simulink model "siso_example_ublf_blf_bs"  (R2021a)
settings: Solver=ode4  StartTime=0.0  StopTime=1.5  FixedStep=0.001  RelTol=1e-3
model workspace (MAT data in the model file):
  scale_start = Simulink.Signal
  scale_start.DataType = 'double'
  scale_start.Dimensions = 1
  scale_start.DimensionsMode = 'auto'
  scale_start.Complexity = 'auto'
  scale_start.SampleTime = 0
  scale_start.SamplingMode = 'auto'
  scale_start.InitialValue = '1'
libraries: simulink x2
settings Model: OrderedModelArguments=off  Creator=14244039  LastModifiedBy=14244039

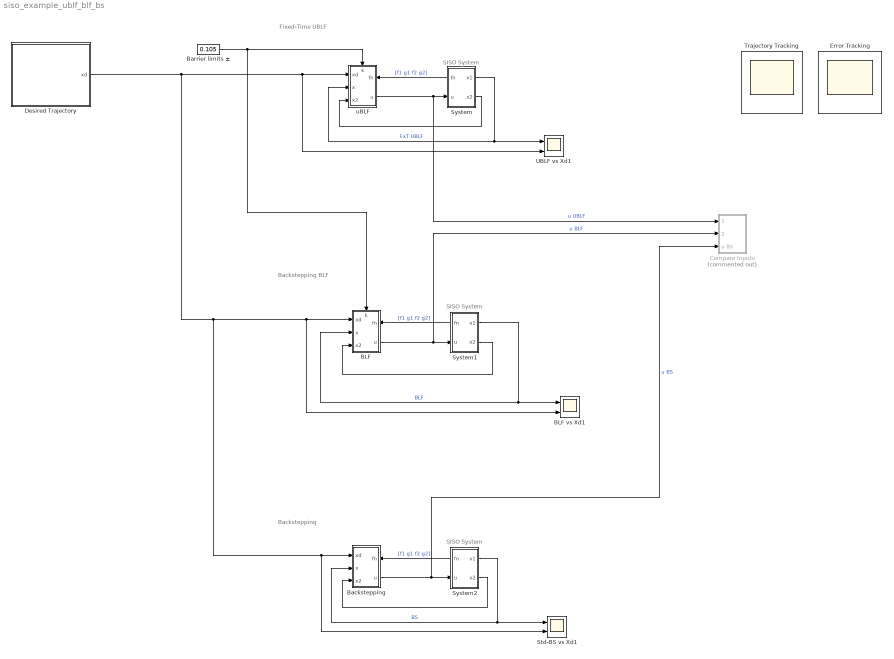
== system siso_example_ublf_blf_bs ==
  note: SISO System
  note: Backstepping
  note: Backstepping BLF
  note: Fixed-Time UBLF
  note: SISO System
  note: SISO System
  BLF : Subsystem
      settings: PortSchema="{\"entries\":[{\"content\":{\"sides\":[{\"content\":{\"connectorIds\":[\"In1\",\"In2\",\"In3\"]},\"type\":\"ConnectorPlacement.EquallySpacedRectSide\",\"uuid\":\"d2f7d382-6195-45e8-bd6d-6d057452a9ba\"},{\"content\":{\"connectorIds\":[\"In5\",\"Out1\"],\"side\":\"RIGHT\"},\"type\":\"ConnectorPlacement.EquallySpacedRectSide\",\"uuid\":\"a1535a06-1066-4f88-a239-6dd18a46e73c\"},{\"content\":{\"connectorIds\":[\"In4\"],\"side\":\"TOP\"},\"type\":\"ConnectorPlacement.EquallySpacedRectSide\",\"uuid\":\"b65ca63e-d25a-45d6-8018-31a25176dac1\"}]},\"type\":\"ConnectorPlacement.EquallySpacedConnector\",\"uuid\":\"280ac837-5d25-45ee-8f8e-187f8883864d\"}],\"packageUris\":[\"http://schema.mathworks.com/mf0/Connector/R2020b\"],\"version\":\"1.0\"}"
  BLF vs Xd1 : Scope  NumInputPorts=2
  Backstepping : Subsystem
      settings: PortSchema="{\"entries\":[{\"content\":{\"sides\":[{\"content\":{\"connectorIds\":[\"In1\",\"In2\",\"In3\"]},\"type\":\"ConnectorPlacement.EquallySpacedRectSide\",\"uuid\":\"d2f7d382-6195-45e8-bd6d-6d057452a9ba\"},{\"content\":{\"connectorIds\":[\"In4\",\"Out1\"],\"side\":\"RIGHT\"},\"type\":\"ConnectorPlacement.EquallySpacedRectSide\",\"uuid\":\"a1535a06-1066-4f88-a239-6dd18a46e73c\"},{\"content\":{\"connectorIds\":[],\"side\":\"TOP\"},\"type\":\"ConnectorPlacement.EquallySpacedRectSide\",\"uuid\":\"b65ca63e-d25a-45d6-8018-31a25176dac1\"}]},\"type\":\"ConnectorPlacement.EquallySpacedConnector\",\"uuid\":\"280ac837-5d25-45ee-8f8e-187f8883864d\"}],\"packageUris\":[\"http://schema.mathworks.com/mf0/Connector/R2020b\"],\"version\":\"1.0\"}"
  Barrier limits ± : Constant  Value=0.105
  Compare Inputs : Subsystem  Commented=on
  Desired Trajectory : Subsystem
  Error Tracking : Scope
      settings: Floating=on
  Std-BS vs Xd1 : Scope  NumInputPorts=2
  System : Subsystem
      settings: PortSchema="{\"entries\":[{\"content\":{\"sides\":[{\"content\":{\"connectorIds\":[\"Out3\",\"In1\"]},\"type\":\"ConnectorPlacement.EquallySpacedRectSide\",\"uuid\":\"44a46657-7d00-4f6d-80a4-fbe778e41b73\"},{\"content\":{\"connectorIds\":[\"Out1\",\"Out2\"],\"side\":\"RIGHT\"},\"type\":\"ConnectorPlacement.EquallySpacedRectSide\",\"uuid\":\"1134a23b-2977-450f-b075-fdef5e2c40fa\"},{\"content\":{\"connectorIds\":[],\"side\":\"TOP\"},\"type\":\"ConnectorPlacement.EquallySpacedRectSide\",\"uuid\":\"dbd99adc-543a-4e22-b7a4-6b9f86b8ed0c\"}]},\"type\":\"ConnectorPlacement.EquallySpacedConnector\",\"uuid\":\"979c4d4e-bab9-42b7-bb8f-441469f19c5c\"}],\"packageUris\":[\"http://schema.mathworks.com/mf0/Connector/R2020b\"],\"version\":\"1.0\"}"
  System1 : Subsystem
      settings: PortSchema="{\"entries\":[{\"content\":{\"sides\":[{\"content\":{\"connectorIds\":[\"Out3\",\"In1\"]},\"type\":\"ConnectorPlacement.EquallySpacedRectSide\",\"uuid\":\"44a46657-7d00-4f6d-80a4-fbe778e41b73\"},{\"content\":{\"connectorIds\":[\"Out1\",\"Out2\"],\"side\":\"RIGHT\"},\"type\":\"ConnectorPlacement.EquallySpacedRectSide\",\"uuid\":\"1134a23b-2977-450f-b075-fdef5e2c40fa\"},{\"content\":{\"connectorIds\":[],\"side\":\"TOP\"},\"type\":\"ConnectorPlacement.EquallySpacedRectSide\",\"uuid\":\"dbd99adc-543a-4e22-b7a4-6b9f86b8ed0c\"}]},\"type\":\"ConnectorPlacement.EquallySpacedConnector\",\"uuid\":\"979c4d4e-bab9-42b7-bb8f-441469f19c5c\"}],\"packageUris\":[\"http://schema.mathworks.com/mf0/Connector/R2020b\"],\"version\":\"1.0\"}"
  System2 : Subsystem
      settings: PortSchema="{\"entries\":[{\"content\":{\"sides\":[{\"content\":{\"connectorIds\":[\"Out3\",\"In1\"]},\"type\":\"ConnectorPlacement.EquallySpacedRectSide\",\"uuid\":\"44a46657-7d00-4f6d-80a4-fbe778e41b73\"},{\"content\":{\"connectorIds\":[\"Out1\",\"Out2\"],\"side\":\"RIGHT\"},\"type\":\"ConnectorPlacement.EquallySpacedRectSide\",\"uuid\":\"1134a23b-2977-450f-b075-fdef5e2c40fa\"},{\"content\":{\"connectorIds\":[],\"side\":\"TOP\"},\"type\":\"ConnectorPlacement.EquallySpacedRectSide\",\"uuid\":\"dbd99adc-543a-4e22-b7a4-6b9f86b8ed0c\"}]},\"type\":\"ConnectorPlacement.EquallySpacedConnector\",\"uuid\":\"979c4d4e-bab9-42b7-bb8f-441469f19c5c\"}],\"packageUris\":[\"http://schema.mathworks.com/mf0/Connector/R2020b\"],\"version\":\"1.0\"}"
  Trajectory Tracking : Scope
      settings: Floating=on
  UBLF vs Xd1 : Scope  NumInputPorts=2
  uBLF : Subsystem
      settings: PortSchema="{\"entries\":[{\"content\":{\"sides\":[{\"content\":{\"connectorIds\":[\"In1\",\"In2\",\"In3\"]},\"type\":\"ConnectorPlacement.EquallySpacedRectSide\",\"uuid\":\"d2f7d382-6195-45e8-bd6d-6d057452a9ba\"},{\"content\":{\"connectorIds\":[\"In5\",\"Out1\"],\"side\":\"RIGHT\"},\"type\":\"ConnectorPlacement.EquallySpacedRectSide\",\"uuid\":\"a1535a06-1066-4f88-a239-6dd18a46e73c\"},{\"content\":{\"connectorIds\":[\"In4\"],\"side\":\"TOP\"},\"type\":\"ConnectorPlacement.EquallySpacedRectSide\",\"uuid\":\"b65ca63e-d25a-45d6-8018-31a25176dac1\"}]},\"type\":\"ConnectorPlacement.EquallySpacedConnector\",\"uuid\":\"280ac837-5d25-45ee-8f8e-187f8883864d\"}],\"packageUris\":[\"http://schema.mathworks.com/mf0/Connector/R2020b\"],\"version\":\"1.0\"}"
  wires:
  System/1(x1) -> uBLF/2(x), UBLF vs Xd1/1  "FxT UBLF"
  System/2(x2) -> uBLF/3(x2)
  System/3(fn) -> uBLF/5(fn)  "[f1 g1 f2 g2]"
  uBLF/1(u) -> Compare Inputs/1(u UBLF), System/1(u)  "u UBLF"
  System1/3(fn) -> BLF/5(fn)  "[f1 g1 f2 g2]"
  BLF/1(u) -> Compare Inputs/2(u ABLF), System1/1(u)  "u BLF"
  System1/1(x1) -> BLF vs Xd1/1, BLF/2(x)  "BLF"
  System1/2(x2) -> BLF/3(x2)
  System2/1(x1) -> Backstepping/2(x), Std-BS vs Xd1/1  "BS"
  System2/2(x2) -> Backstepping/3(x2)
  Desired Trajectory/1(xd) -> uBLF/1(xd), UBLF vs Xd1/2, BLF/1(xd), BLF vs Xd1/2, Std-BS vs Xd1/2, Backstepping/1(xd)
  System2/3(fn) -> Backstepping/4(fn)  "[f1 g1 f2 g2]"
  Backstepping/1(u) -> Compare Inputs/3(u BS), System2/1(u)  "u BS"
  Barrier limits ±/1 -> BLF/4(k), uBLF/4(k)

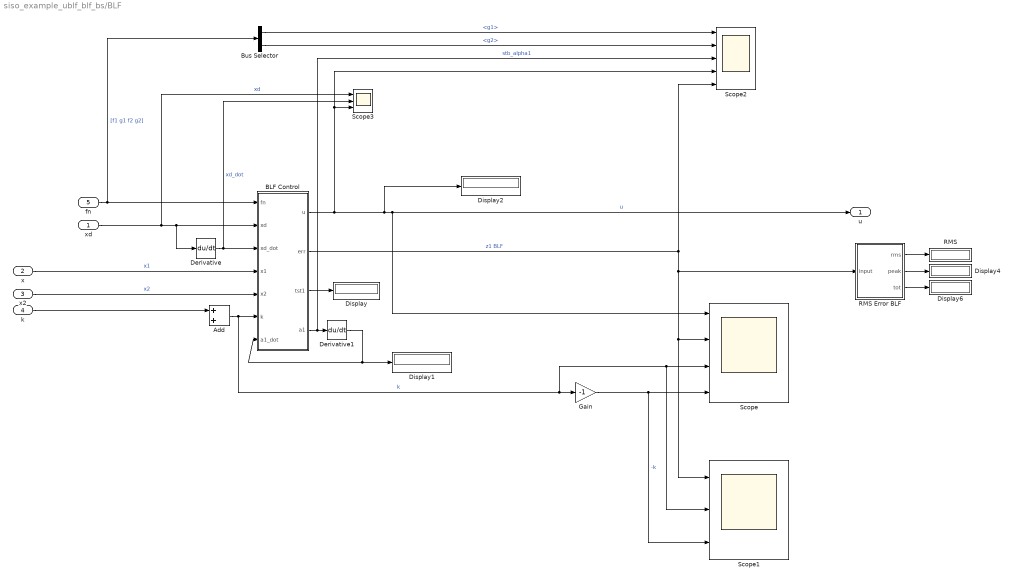
== system siso_example_ublf_blf_bs/BLF ==
  xd : Inport
  x : Inport  Port=2
  x2 : Inport  Port=3
  k : Inport  Port=4
  fn : Inport  Port=5
  Add : Sum
  BLF Control : MATLAB Function  TreatAsAtomicUnit=on
  Bus Selector : BusSelector  OutputSignals=g1,g2
  Derivative : Derivative
  Derivative1 : Derivative
  Display{,1..2,4,6} (5 alike) : Display
  Gain : Gain  Gain=-1
  RMS : Display
  RMS Error BLF : MATLAB Function  TreatAsAtomicUnit=on
  Scope : Scope  NumInputPorts=4
  Scope1 : Scope  NumInputPorts=3
  Scope2 : Scope  NumInputPorts=5
  Scope3 : Scope  NumInputPorts=3
  u : Outport
  wires:
  Bus Selector/2 -> Scope2/2  "<g2>"
  Bus Selector/1 -> Scope2/1  "<g1>"
  fn/1 -> BLF Control/1(fn), Bus Selector/1  "[f1 g1 f2 g2]"
  Gain/1 -> Scope/4, Scope1/3  "-k"
  Add/1 -> BLF Control/6(k), Gain/1, Scope/3, Scope1/2  "k"
  k/1 -> Add/1
  BLF Control/1(u) -> Scope3/3, Scope2/4, Display2/1, Scope/1, u/1  "u"
  BLF Control/4(a1) -> Derivative1/1, Scope2/3  "stb_alpha1"
  xd/1 -> BLF Control/2(xd), Derivative/1, Scope3/1  "xd"
  x2/1 -> BLF Control/5(x2)  "x2"
  Derivative1/1 -> Display1/1, BLF Control/7(a1_dot)
  BLF Control/3(tst1) -> Display/1
  BLF Control/2(err) -> Scope2/5, RMS Error BLF/1(input), Scope/2, Scope1/1  "z1 BLF"
  x/1 -> BLF Control/4(x1)  "x1"
  Derivative/1 -> BLF Control/3(xd_dot), Scope3/2  "xd_dot"
  RMS Error BLF/1(rms) -> RMS/1
  RMS Error BLF/3(tot) -> Display6/1
  RMS Error BLF/2(peak) -> Display4/1

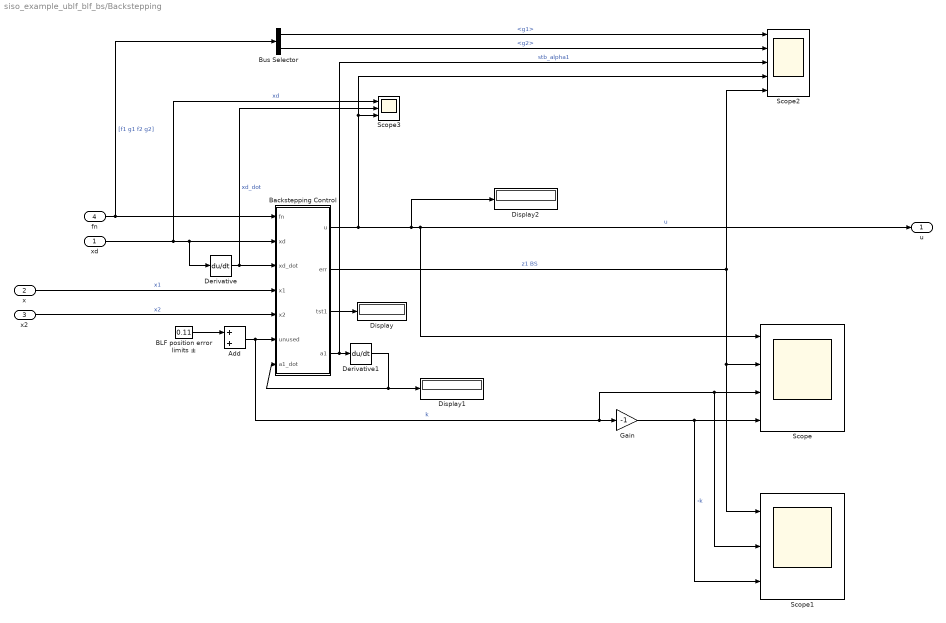
== system siso_example_ublf_blf_bs/Backstepping ==
  xd : Inport
  x : Inport  Port=2
  x2 : Inport  Port=3
  fn : Inport  Port=4
  Add : Sum
  BLF position error limits ± : Constant  Value=0.11
  Backstepping Control : MATLAB Function  TreatAsAtomicUnit=on
  Bus Selector : BusSelector  OutputSignals=g1,g2
  Derivative : Derivative
  Derivative1 : Derivative
  Display : Display
  Display1 : Display
  Display2 : Display
  Gain : Gain  Gain=-1
  Scope : Scope  NumInputPorts=4
  Scope1 : Scope  NumInputPorts=3
  Scope2 : Scope  NumInputPorts=5
  Scope3 : Scope  NumInputPorts=3
  u : Outport
  wires:
  Bus Selector/2 -> Scope2/2  "<g2>"
  Bus Selector/1 -> Scope2/1  "<g1>"
  fn/1 -> Backstepping Control/1(fn), Bus Selector/1  "[f1 g1 f2 g2]"
  Gain/1 -> Scope/4, Scope1/3  "-k"
  Add/1 -> Backstepping Control/6(unused), Gain/1, Scope/3, Scope1/2  "k"
  BLF position error limits ±/1 -> Add/1
  Backstepping Control/1(u) -> Scope3/3, Scope2/4, Display2/1, Scope/1, u/1  "u"
  Backstepping Control/4(a1) -> Derivative1/1, Scope2/3  "stb_alpha1"
  xd/1 -> Backstepping Control/2(xd), Derivative/1, Scope3/1  "xd"
  x2/1 -> Backstepping Control/5(x2)  "x2"
  Derivative1/1 -> Display1/1, Backstepping Control/7(a1_dot)
  Backstepping Control/3(tst1) -> Display/1
  Backstepping Control/2(err) -> Scope2/5, Scope/2, Scope1/1  "z1 BS"
  x/1 -> Backstepping Control/4(x1)  "x1"
  Derivative/1 -> Backstepping Control/3(xd_dot), Scope3/2  "xd_dot"

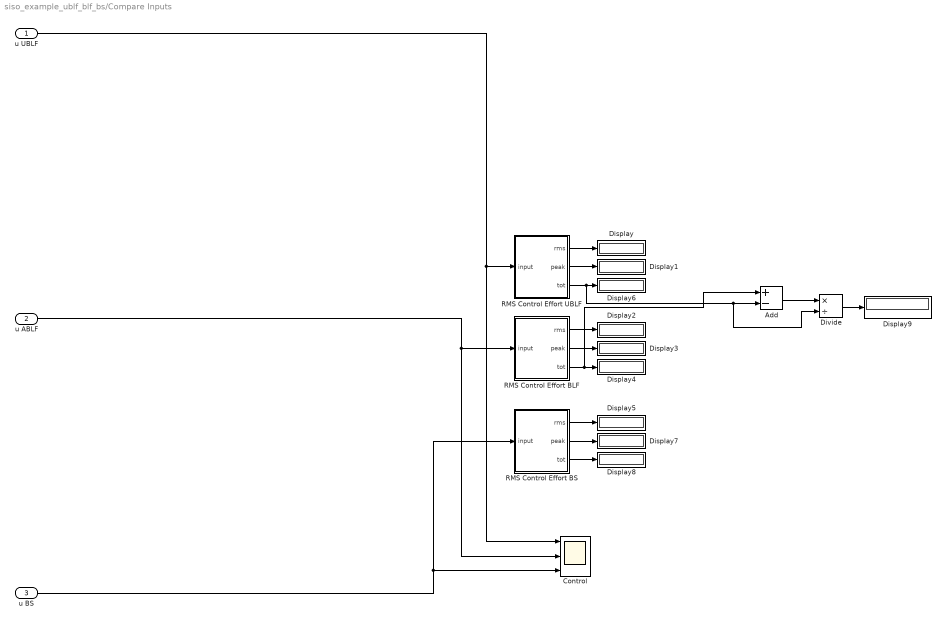
== system siso_example_ublf_blf_bs/Compare Inputs ==
  u UBLF : Inport
  u ABLF : Inport  Port=2
  u BS : Inport  Port=3
  Add : Sum  Inputs=+-
  Control : Scope  NumInputPorts=3
  Display{,1..9} (10 alike) : Display
  Divide : Product  Inputs=*/
  RMS Control Effort BLF : MATLAB Function  TreatAsAtomicUnit=on
  RMS Control Effort BS : MATLAB Function  TreatAsAtomicUnit=on
  RMS Control Effort UBLF : MATLAB Function  TreatAsAtomicUnit=on
  wires:
  RMS Control Effort BS/2(peak) -> Display7/1
  RMS Control Effort BS/3(tot) -> Display8/1
  u ABLF/1 -> RMS Control Effort BLF/1(input), Control/2
  RMS Control Effort BLF/2(peak) -> Display3/1
  u UBLF/1 -> Control/1, RMS Control Effort UBLF/1(input)
  RMS Control Effort UBLF/2(peak) -> Display1/1
  RMS Control Effort UBLF/1(rms) -> Display/1
  RMS Control Effort BLF/1(rms) -> Display2/1
  RMS Control Effort BLF/3(tot) -> Add/1, Display4/1
  RMS Control Effort BS/1(rms) -> Display5/1
  u BS/1 -> RMS Control Effort BS/1(input), Control/3
  Divide/1 -> Display9/1
  RMS Control Effort UBLF/3(tot) -> Divide/2, Add/2, Display6/1
  Add/1 -> Divide/1

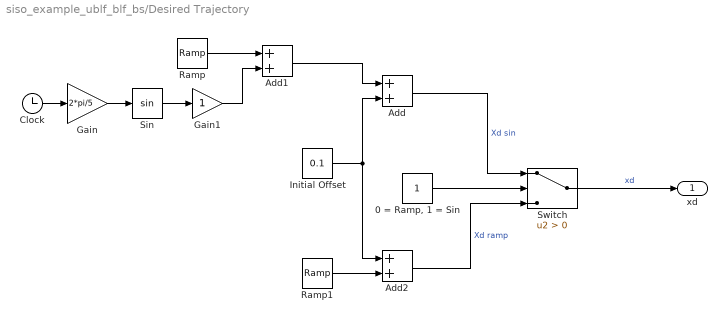
== system siso_example_ublf_blf_bs/Desired Trajectory ==
  "0 = Ramp, 1 = Sin" : Constant
  Add : Sum
  Add1 : Sum
  Add2 : Sum
  Clock : Clock
  Gain : Gain  Gain=2*pi/5
  Gain1 : Gain
  Initial Offset : Constant  Value=0.1
  Ramp : simulink/Sources/Ramp  slope=1  start=0  InitialOutput=0
  Ramp1 : simulink/Sources/Ramp  slope=0.2  start=0  InitialOutput=0
  Sin : Trigonometry
  Switch : Switch  Criteria=u2 > Threshold
  xd : Outport
  wires:
  Gain1/1 -> Add1/2
  Ramp1/1 -> Add2/2
  Sin/1 -> Gain1/1
  Clock/1 -> Gain/1
  Ramp/1 -> Add1/1
  Gain/1 -> Sin/1
  Add/1 -> Switch/1  "Xd sin"
  Initial Offset/1 -> Add/2, Add2/1
  Add1/1 -> Add/1
  "0 = Ramp, 1 = Sin"/1 -> Switch/2
  Add2/1 -> Switch/3  "Xd ramp"
  Switch/1 -> xd/1  "xd"

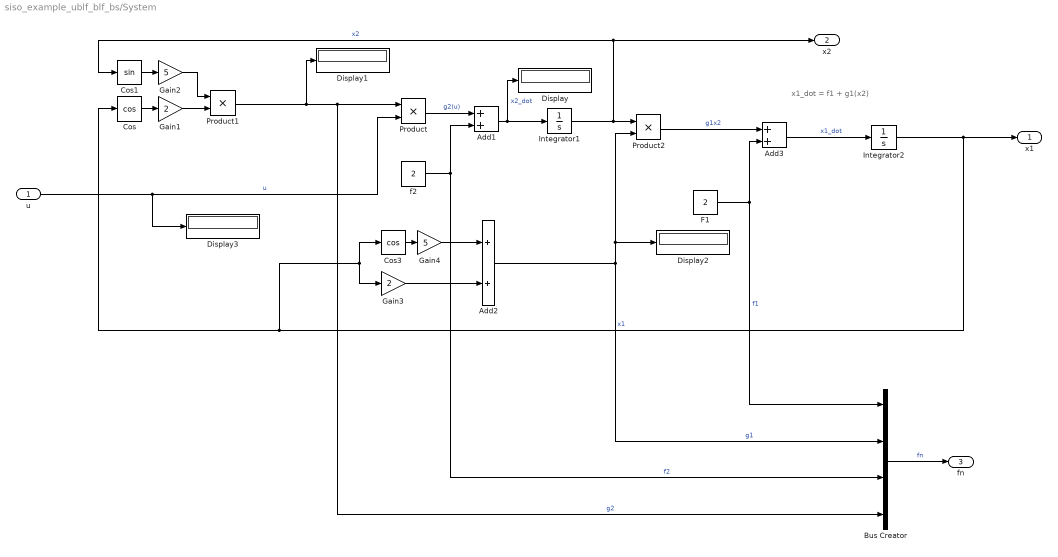
== system siso_example_ublf_blf_bs/System ==
  note: x1_dot = f1 + g1(x2)
  u : Inport
  Add1 : Sum
  Add2 : Sum
  Add3 : Sum
  Bus Creator : BusCreator  Inputs=4
  Cos : Trigonometry  Operator=cos
  Cos1 : Trigonometry
  Cos3 : Trigonometry  Operator=cos
  Display{,1..3} (4 alike) : Display
  F1 : Constant  Value=2
  Gain1 : Gain  Gain=2
  Gain2 : Gain  Gain=5
  Gain3 : Gain  Gain=2
  Gain4 : Gain  Gain=5
  Integrator1 : Integrator  InitialCondition=0.01  IgnoreLimit=on
  Integrator2 : Integrator
  Product : Product
  Product1 : Product
  Product2 : Product
  f2 : Constant  Value=2
  x1 : Outport
  x2 : Outport  Port=2
  fn : Outport  Port=3  PortDimensions=4
  wires:
  u/1 -> Display3/1, Product/2  "u"
  Integrator1/1 -> x2/1, Cos1/1, Product2/1  "x2"
  Add1/1 -> Display/1, Integrator1/1  "x2_dot"
  Product/1 -> Add1/1  "g2(u)"
  Integrator2/1 -> x1/1, Gain3/1, Cos3/1, Cos/1  "x1"
  F1/1 -> Add3/2, Bus Creator/1  "f1"
  Bus Creator/1 -> fn/1  "fn"
  Gain1/1 -> Product1/2
  Cos/1 -> Gain1/1
  Cos1/1 -> Gain2/1
  Gain2/1 -> Product1/1
  f2/1 -> Bus Creator/3, Add1/2  "f2"
  Gain4/1 -> Add2/1
  Cos3/1 -> Gain4/1
  Gain3/1 -> Add2/2
  Product2/1 -> Add3/1  "g1x2"
  Product1/1 -> Display1/1, Bus Creator/4, Product/1  "g2"
  Add2/1 -> Bus Creator/2, Display2/1, Product2/2  "g1"
  Add3/1 -> Integrator2/1  "x1_dot"

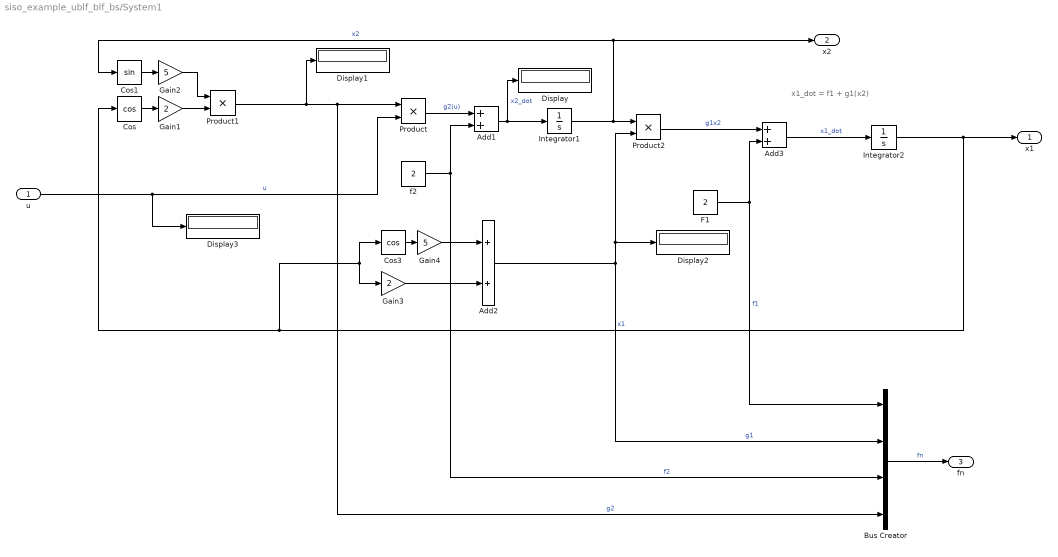
== system siso_example_ublf_blf_bs/System1 ==
  note: x1_dot = f1 + g1(x2)
  u : Inport
  Add1 : Sum
  Add2 : Sum
  Add3 : Sum
  Bus Creator : BusCreator  Inputs=4
  Cos : Trigonometry  Operator=cos
  Cos1 : Trigonometry
  Cos3 : Trigonometry  Operator=cos
  Display{,1..3} (4 alike) : Display
  F1 : Constant  Value=2
  Gain1 : Gain  Gain=2
  Gain2 : Gain  Gain=5
  Gain3 : Gain  Gain=2
  Gain4 : Gain  Gain=5
  Integrator1 : Integrator  InitialCondition=0.01  IgnoreLimit=on
  Integrator2 : Integrator
  Product : Product
  Product1 : Product
  Product2 : Product
  f2 : Constant  Value=2
  x1 : Outport
  x2 : Outport  Port=2
  fn : Outport  Port=3  PortDimensions=4
  wires:
  Add3/1 -> Integrator2/1  "x1_dot"
  Add2/1 -> Product2/2, Display2/1, Bus Creator/2  "g1"
  Product1/1 -> Product/1, Bus Creator/4, Display1/1  "g2"
  Product2/1 -> Add3/1  "g1x2"
  Gain3/1 -> Add2/2
  Cos3/1 -> Gain4/1
  Gain4/1 -> Add2/1
  f2/1 -> Add1/2, Bus Creator/3  "f2"
  Gain2/1 -> Product1/1
  Cos1/1 -> Gain2/1
  Cos/1 -> Gain1/1
  Gain1/1 -> Product1/2
  Bus Creator/1 -> fn/1  "fn"
  F1/1 -> Bus Creator/1, Add3/2  "f1"
  Integrator2/1 -> Cos/1, Cos3/1, Gain3/1, x1/1  "x1"
  Product/1 -> Add1/1  "g2(u)"
  Add1/1 -> Integrator1/1, Display/1  "x2_dot"
  Integrator1/1 -> Product2/1, Cos1/1, x2/1  "x2"
  u/1 -> Product/2, Display3/1  "u"

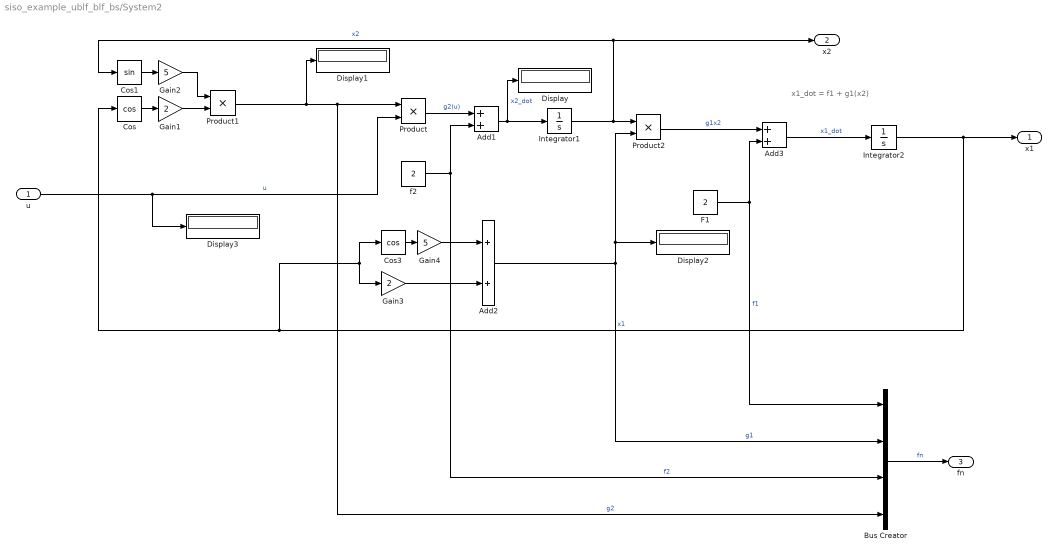
== system siso_example_ublf_blf_bs/System2 ==
  note: x1_dot = f1 + g1(x2)
  u : Inport
  Add1 : Sum
  Add2 : Sum
  Add3 : Sum
  Bus Creator : BusCreator  Inputs=4
  Cos : Trigonometry  Operator=cos
  Cos1 : Trigonometry
  Cos3 : Trigonometry  Operator=cos
  Display{,1..3} (4 alike) : Display
  F1 : Constant  Value=2
  Gain1 : Gain  Gain=2
  Gain2 : Gain  Gain=5
  Gain3 : Gain  Gain=2
  Gain4 : Gain  Gain=5
  Integrator1 : Integrator  InitialCondition=0.01  IgnoreLimit=on
  Integrator2 : Integrator
  Product : Product
  Product1 : Product
  Product2 : Product
  f2 : Constant  Value=2
  x1 : Outport
  x2 : Outport  Port=2
  fn : Outport  Port=3  PortDimensions=4
  wires:
  u/1 -> Display3/1, Product/2  "u"
  Integrator1/1 -> x2/1, Cos1/1, Product2/1  "x2"
  Add1/1 -> Display/1, Integrator1/1  "x2_dot"
  Product/1 -> Add1/1  "g2(u)"
  Integrator2/1 -> x1/1, Gain3/1, Cos3/1, Cos/1  "x1"
  F1/1 -> Add3/2, Bus Creator/1  "f1"
  Bus Creator/1 -> fn/1  "fn"
  Gain1/1 -> Product1/2
  Cos/1 -> Gain1/1
  Cos1/1 -> Gain2/1
  Gain2/1 -> Product1/1
  f2/1 -> Bus Creator/3, Add1/2  "f2"
  Gain4/1 -> Add2/1
  Cos3/1 -> Gain4/1
  Gain3/1 -> Add2/2
  Product2/1 -> Add3/1  "g1x2"
  Product1/1 -> Display1/1, Bus Creator/4, Product/1  "g2"
  Add2/1 -> Bus Creator/2, Display2/1, Product2/2  "g1"
  Add3/1 -> Integrator2/1  "x1_dot"

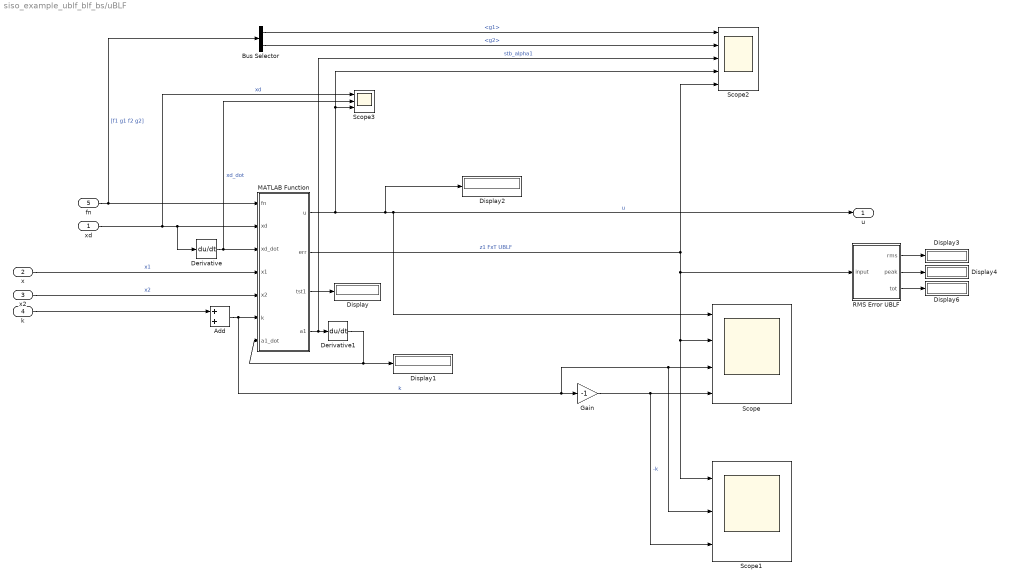
== system siso_example_ublf_blf_bs/uBLF ==
  xd : Inport
  x : Inport  Port=2
  x2 : Inport  Port=3
  k : Inport  Port=4
  fn : Inport  Port=5
  Add : Sum
  Bus Selector : BusSelector  OutputSignals=g1,g2
  Derivative : Derivative
  Derivative1 : Derivative
  Display{,1..4,6} (6 alike) : Display
  Gain : Gain  Gain=-1
  MATLAB Function : MATLAB Function  TreatAsAtomicUnit=on
  RMS Error UBLF : MATLAB Function  TreatAsAtomicUnit=on
  Scope : Scope  NumInputPorts=4
  Scope1 : Scope  NumInputPorts=3
  Scope2 : Scope  NumInputPorts=5
  Scope3 : Scope  NumInputPorts=3
  u : Outport
  wires:
  Derivative/1 -> Scope3/2, MATLAB Function/3(xd_dot)  "xd_dot"
  x/1 -> MATLAB Function/4(x1)  "x1"
  MATLAB Function/2(err) -> RMS Error UBLF/1(input), Scope1/1, Scope/2, Scope2/5  "z1 FxT UBLF"
  MATLAB Function/3(tst1) -> Display/1
  Derivative1/1 -> MATLAB Function/7(a1_dot), Display1/1
  x2/1 -> MATLAB Function/5(x2)  "x2"
  xd/1 -> Scope3/1, Derivative/1, MATLAB Function/2(xd)  "xd"
  MATLAB Function/4(a1) -> Scope2/3, Derivative1/1  "stb_alpha1"
  MATLAB Function/1(u) -> u/1, Scope/1, Display2/1, Scope2/4, Scope3/3  "u"
  k/1 -> Add/1
  Add/1 -> Scope1/2, Scope/3, Gain/1, MATLAB Function/6(k)  "k"
  Gain/1 -> Scope1/3, Scope/4  "-k"
  fn/1 -> Bus Selector/1, MATLAB Function/1(fn)  "[f1 g1 f2 g2]"
  Bus Selector/1 -> Scope2/1  "<g1>"
  Bus Selector/2 -> Scope2/2  "<g2>"
  RMS Error UBLF/3(tot) -> Display6/1
  RMS Error UBLF/2(peak) -> Display4/1
  RMS Error UBLF/1(rms) -> Display3/1

== matlab function siso_example_ublf_blf_bs/Compare Inputs/RMS Control Effort UBLF ==
  settings: updateMethod=DISCRETE
  data: rms output; input input; peak output; tot output
function [rms, peak, tot]  = fcn(input)

persistent total pk t
if isempty(total)
    total = 0;
    pk = 0;
    t = 0;
end

persistent i
if isempty(i)
    i = 0;
end

i=i+1;

if abs(input) > pk
   pk = abs(input); 
end


total = total + (input.^2);

t = t + abs(input);

rms1 = (sqrt(total)) / i;

rms = rms1;
peak = pk;
tot = t;

== matlab function siso_example_ublf_blf_bs/Compare Inputs/RMS Control Effort BLF ==
  settings: updateMethod=DISCRETE
  data: rms output; input input; peak output; tot output
function [rms, peak, tot]  = fcn(input)

persistent total pk t
if isempty(total)
    total = 0;
    pk = 0;
    t = 0;
end

persistent i
if isempty(i)
    i = 0;
end

i=i+1;

if abs(input) > pk
   pk = abs(input); 
end


total = total + (input.^2);

t = t + abs(input);

rms1 = (sqrt(total)) / i;

rms = rms1;
peak = pk;
tot = t;

== matlab function siso_example_ublf_blf_bs/uBLF/MATLAB Function ==
  data: fn input; xd input; u output; xd_dot input; x1 input; x2 input; err output; k input; tst1 output; a1_dot input; a1 output
function [u, err, tst1, a1]   = fcn(fn, xd, xd_dot, x1, x2, k, a1_dot)

%tst1 = zeros(1,2);

% fixed time parameters
    a = 10;
    b = 10;
    a2 = 10;
    b2 = 10;
    
    kpa1 = min(a,a2);
    kpa2 = min(b,b2);
    
    tmax = 5.867/kpa1 + 1/kpa2;

    eps10 = 0.0001;
    eps20 = 0.0001;

% functions from system
    f1 = fn(1); 
    g1 = fn(2);
    f2 = fn(3);
    g2 = fn(4);

    eps1 = 0.00001;
    eps2 = 0.00001;

    z1 = x1 - xd;

    n = ( (k^2) * z1 ) / ( k^2 - ((z1)^2) );
    w = ( (k^2) * (k^2 + (z1)^2) ) / ( ( k^2 - ( (z1)^2 ) )^2 );

%Sn switched when n < eps10
    if abs(n) < eps10
        %Sn = ( (n)^2 )^(3/4);
        Sn = 1.25*( (n)^2 )*( (eps10^2)^(-1/4)) + (-0.25)*( ((n)^2)^2 )*( (eps10^2)^(-5/4));
    else
        Sn = ( (n)^2 )^(3/4);
    end
      
    alp1_hat = ( -(w*xd_dot) + ( a* ( (0.5)^(3/4) ) * ( n/((n)^2) )* Sn ) + ( b * ((0.5)^2)*n*((n)^2) ) );

    stb_alpha1 = -(1/g1)* (( (n*w)*((alp1_hat/w)^2)) / sqrt( ((n*w))^2 * (((alp1_hat/w))^2) + (eps1)^2) +f1 );

    z2 = x2 - stb_alpha1;

   % V1 = 0.5*n^2;
    %V2 = V1 + 0.5*(z2^2);
    
% second step, control input

    %S2 switched when z2 < eps20
    if abs(z2) < eps20
        %S2 = ( (z2)^2 )^(3/4);
        S2 = 1.25*( (z2)^2 )*( (eps20^2)^(-1/4)) + (-0.25)*( ((z2)^2)^2 )*( (eps20^2)^(-5/4));
    else
        S2 = ( (z2)^2 )^(3/4);
    end

    alp2_hat = -a1_dot + ( 0.5^(3/4) * a2 * (z2/( (z2)^2)) * S2 ) + ( ((0.5)^2) * b2 * z2 * (z2^2) ); 
    
    ctl = -(1/g2)*( ((z2 * (alp2_hat)^2) / ( sqrt( ((z2)^2 * (alp2_hat)^2 + eps2^2) )  ) ) + n*w*g1 + f2  );

% if fxt == 1
%     Tmax = 1/(a*(1-gma)) + 1/b*(beta-1); % if fixed time selected calculate max convergence time
% else
%      Tmax = 0; % 
% end;


u = ctl;
err = z1;
tst1 = tmax;
a1 = stb_alpha1;

== matlab function siso_example_ublf_blf_bs/BLF/BLF Control ==
  data: fn input; xd input; u output; xd_dot input; x1 input; x2 input; err output; k input; tst1 output; a1_dot input; a1 output
function [u, err, tst1, a1]   = fcn(fn, xd, xd_dot, x1, x2, k, a1_dot)


% controller gains
a1  = 10;
a2  = 10;



% functions from system
    f1  = fn(1); 
    g1  = fn(2);
    f2  = fn(3);
    g2  = fn(4);

    z1  = x1 - xd;

    w   = k^2 - z1^2;
    
    alpha1  = (1/g1)*(-f1 -w*a1*z1 + xd_dot);
    
    z2  = x2-alpha1;
    
    ctl = (1/g2)*(-f2 + a1_dot - a2*z2 - (g1*z1)/w);


u = ctl;
err = z1;
tst1 = 0;
a1 = alpha1;

== matlab function siso_example_ublf_blf_bs/Backstepping/Backstepping Control ==
  data: fn input; xd input; u output; xd_dot input; x1 input; x2 input; err output; unused input; tst1 output; a1_dot input; a1 output
function [u, err, tst1, a1]   = fcn(fn, xd, xd_dot, x1, x2, ~, a1_dot)


% controller gains
a1  = 5;
a2  = 10;

% functions from system
    f1  = fn(1); 
    g1  = fn(2);
    f2  = fn(3);
    g2  = fn(4);

    z1  = x1 - xd;
    
    alpha1  = (1/g1)*(-f1 -a1*z1 + xd_dot);
    
    z2  = x2-alpha1;
    
    ctl = (1/g2)*(-f2 + a1_dot - a2*z2 -g1*z1);


u = ctl;
err = z1;
tst1 = 0;
a1 = alpha1;

== matlab function siso_example_ublf_blf_bs/Compare Inputs/RMS Control Effort BS ==
  settings: updateMethod=DISCRETE
  data: rms output; input input; peak output; tot output
function [rms, peak, tot]  = fcn(input)

persistent total pk t
if isempty(total)
    total = 0;
    pk = 0;
    t = 0;
end

persistent i
if isempty(i)
    i = 0;
end

i=i+1;

if abs(input) > pk
   pk = abs(input); 
end


total = total + (input.^2);

t = t + abs(input);

rms1 = (sqrt(total)) / i;

rms = rms1;
peak = pk;
tot = t;

== matlab function siso_example_ublf_blf_bs/uBLF/RMS Error UBLF ==
  settings: updateMethod=DISCRETE
  data: rms output; input input; peak output; tot output
function [rms, peak, tot]  = fcn(input)

persistent total pk t
if isempty(total)
    total = 0;
    pk = 0;
    t = 0;
end

persistent i
if isempty(i)
    i = 0;
end

i=i+1;

if abs(input) > pk
   pk = abs(input); 
end


total = total + (input.^2);

t = t + abs(input);

rms1 = (sqrt(total)) / i;

rms = rms1;
peak = pk;
tot = t;

== matlab function siso_example_ublf_blf_bs/BLF/RMS Error BLF ==
  settings: updateMethod=DISCRETE
  data: rms output; input input; peak output; tot output
function [rms, peak, tot]  = fcn(input)

persistent total pk t
if isempty(total)
    total = 0;
    pk = 0;
    t = 0;
end

persistent i
if isempty(i)
    i = 0;
end

i=i+1;

if abs(input) > pk
   pk = abs(input); 
end


total = total + (input.^2);

t = t + abs(input);

rms1 = (sqrt(total)) / i;

rms = rms1;
peak = pk;
tot = t;
